simulink model "exercise_3sim"  (R2025b)
settings: Solver=VariableStepAuto  StartTime=0.0  StopTime=10  RelTol=1e-3
values from neighbouring files (symbols this model uses):
  I_c = 0.3    [exercise_3.m]
  K = 25000    [Exercise1.m]    (also in Exercise_2.m; exercise_3.m)
  K_p = 0    [exercise_3.m]
  ms = 400    [Exercise1.m]    (also in Exercise_2.m; exercise_3.m)
  mu = 50    [Exercise1.m]    (also in Exercise_2.m; exercise_3.m)
  P = 150000    [Exercise1.m]    (also in Exercise_2.m; exercise_3.m)
undefined symbols (not defined in the file or in its folder): sigbuilder_block
settings Model: Creator=carlonovara  LastModifiedBy=denni
settings SolverCC: AlgebraicLoopSolver=TrustRegion
settings DataIOCC: ReturnWorkspaceOutputs=off
settings DebuggingCC: UnconnectedInputMsg=warning  UnconnectedOutputMsg=warning  UnconnectedLineMsg=warning
settings ModelReferenceCC: EnableRefExpFcnMdlSchedulingChecks=on
settings RTWCC: GPUComputeCapability=3.5  DLArmComputeVersion=19.05

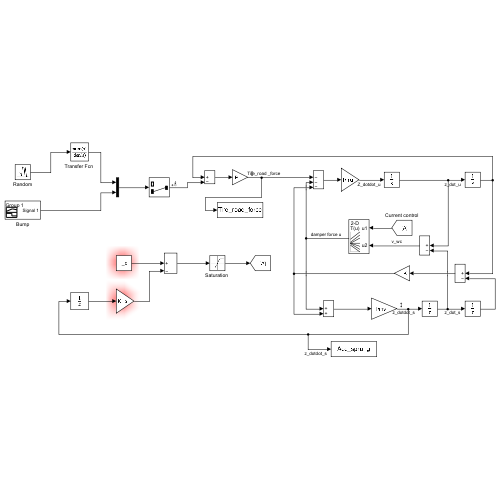
[thumbnail: Simulink's stored preview of the top-level diagram]
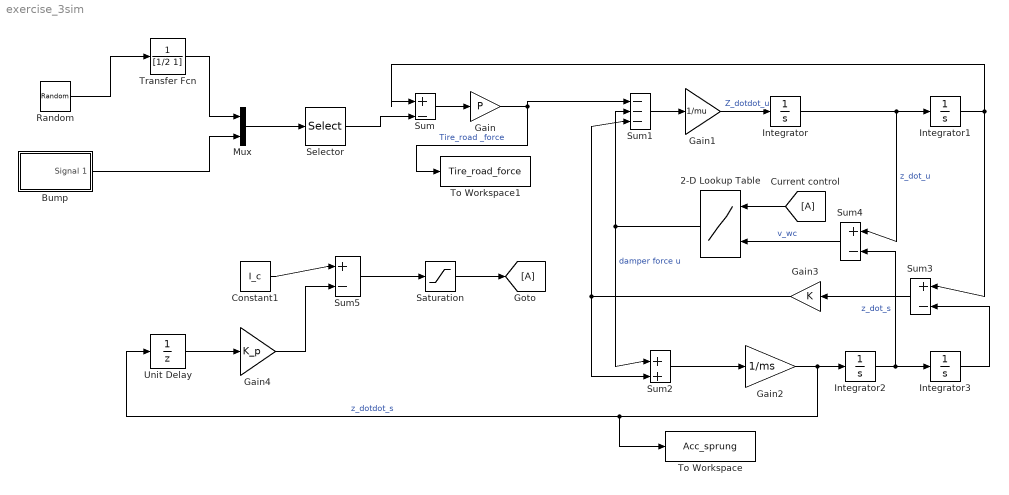
== system exercise_3sim ==
  2-D Lookup Table : Lookup_n-D  LookupTableObject=''  BreakpointsForDimension1=[0.29; 1.6]  BreakpointsForDimension2=[-1.5 -0.6 -0.1 0 0.1 0.6 1.5]  BreakpointsForDimension1FirstPoint=10  BreakpointsForDimension2FirstPoint=10  BreakpointsForDimension1Spacing=12  BreakpointsForDimension2Spacing=12  IndexSearchMethod=Linear search  Table=[-1050 -250 -50 0 50 400 1750;-3900 -2800 -1300 0 2200 3700 5000]  DiagnosticForOutOfRangeInput=Error  InternalRulePriority=Speed  RndMeth=Simplest
      settings: InputPortMap=u0,u1
  Bump : Subsystem  Tag=STV Subsys  LoadFcn=sigbuilder_block('load');  StartFcn=sigbuilder_block('start');  StopFcn=sigbuilder_block('stop');  ClipboardFcn=sigbuilder_block('clipboard');  mask(Sigbuilder block){tuvar=[0:10]}
      mask help: Simulink:masks:SigbuilderBlock_MD
      mask init:
      | if ~strcmp(get_param(bdroot(gcbh),'SimulationStatus'),'stopped') tuvar = sigbuilder_block('maskInit'); end
      settings: CopyFcn=sigbuilder_block('copy');  DeleteFcn=sigbuilder_block('delete');  ModelCloseFcn=sigbuilder_block('modelClose');  PreSaveFcn=sigbuilder_block('preSave');  PauseFcn=sigbuilder_block('pause');  ContinueFcn=sigbuilder_block('continue');  NameChangeFcn=sigbuilder_block('namechange');  OpenFcn=sigbuilder_block('open',[252.75 107.25 644.25 387.75 ]);  CloseFcn=sigbuilder_block('close');
      mask Display: plot(0, 0, 100, 100,[2, 2, 32, 32, 2], [68, 8, 8, 68, 68],[32, 2], [38, 38], [32, 19, 2],[53, 60, 44], [32, 17, 17, 2],[16, 16, 31, 31]);txt = getActiveGroup(gcbh);text(2, 100, txt,'verticalAlignment', 'top');
  Constant1 : Constant  Value=I_c
  Current control : From
  Gain : Gain  Gain=P
  Gain1 : Gain  Gain=1/mu
  Gain2 : Gain  Gain=1/ms
  Gain3 : Gain  Gain=K
  Gain4 : Gain  Gain=K_p
  Goto : Goto
  Integrator{,1..3} (4 alike) : Integrator
  Mux : Mux  Inputs=2
  Random : RandomNumber  Variance=0.05^2  Seed=4521  SampleTime=0.02
  "Saturation " : Saturate  UpperLimit=1.6  LowerLimit=0.29
  Selector : Selector  InputPortWidth=2  IndexOptions=Index vector (dialog)  Indices=inp  OutputSizes=1
  Sum{,3..5} (4 alike) : Sum  Inputs=|+-
  Sum1 : Sum  Inputs=|---
  Sum2 : Sum  Inputs=|++
  To Workspace : ToWorkspace  VariableName=Acc_sprung  SampleTime=-1
  To Workspace1 : ToWorkspace  VariableName=Tire_road_force  SampleTime=-1
  "Transfer Fcn " : TransferFcn  Denominator=[1/2 1]
  Unit Delay : UnitDelay  SampleTime=0.005  HasFrameUpgradeWarning=on
  wires:
  Bump/1(Signal 1) -> Mux/2
  Random/1 -> "Transfer Fcn "/1
  "Transfer Fcn "/1 -> Mux/1
  "Saturation "/1 -> Goto/1
  2-D Lookup Table/1 -> Sum1/2, Sum2/1  "damper force u"
  Gain3/1 -> Sum1/3, Sum2/2
  Gain1/1 -> Integrator/1  "Z_dotdot_u"
  Current control/1 -> 2-D Lookup Table/1
  Integrator/1 -> Sum4/1, Integrator1/1  "z_dot_u"
  Selector/1 -> Sum/2
  Unit Delay/1 -> Gain4/1
  Sum4/1 -> 2-D Lookup Table/2  "v_wc"
  Sum1/1 -> Gain1/1
  Integrator1/1 -> Sum3/1, Sum/1
  Integrator3/1 -> Sum3/2
  Gain4/1 -> Sum5/2
  Constant1/1 -> Sum5/1
  Sum/1 -> Gain/1
  Sum2/1 -> Gain2/1
  Integrator2/1 -> Sum4/2, Integrator3/1  "z_dot_s"
  Gain/1 -> To Workspace1/1, Sum1/1  "Tire_road _force"
  Sum5/1 -> "Saturation "/1
  Gain2/1 -> To Workspace/1, Unit Delay/1, Integrator2/1  "z_dotdot_s"
  Sum3/1 -> Gain3/1
  Mux/1 -> Selector/1

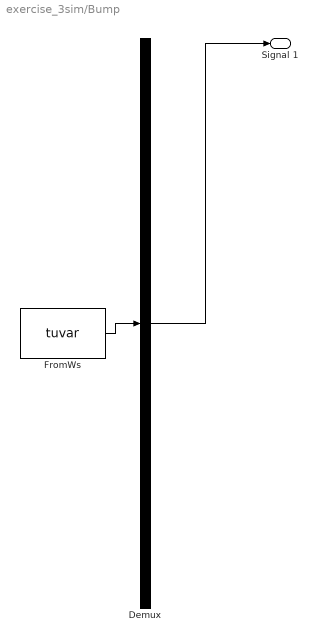
== system exercise_3sim/Bump ==
  Demux : Demux  Tag=STV Demux  Outputs=1
      settings: DisplayOption=none
  FromWs : FromWorkspace  Tag=STV FromWs  VariableName=tuvar
      SigBuilderData=|
      | common.afterFinalStr = 'Extrapolate'
      | common.sampleTime = 0
      | dataSet.timeRange = [0 10]
      | dataSet.name = 'Group 1'
      | sbobj.Groups.Name = 'Group 1'
      | sbobj.Groups.Signals.Name = 'Signal 1'
      | sbobj.Groups.Signals.XData = [0 3.2 3.5 4.5 4.8 10]
      | sbobj.Groups.Signals.YData = [0 0 0.08 0.08 0 0]
  Signal 1 : Outport  Tag=STV Outport
  wires:
  Demux/1 -> Signal 1/1
  FromWs/1 -> Demux/1
